simulink model "MPC_sim_sol"  (R2023b)
settings: Solver=FixedStepDiscrete  StartTime=0.0  StopTime=40  FixedStep=1  RelTol=1e-3
values from neighbouring files (symbols this model uses):
  A = [ 0 , 1 ; 0 , 0 ]    [FDBlin_pend_par_sol.m]    (also in MPC_par_sol.m = [ 1 1 ; 0 1 ]; MPC_sol.m = [ 1 1 ; 0 1 ])
  B = [ 0 ; 1 ]    [FDBlin_pend_par_sol.m]    (also in MPC_par_sol.m; MPC_sol.m)
  H = 2*(Bb'*Qb*Bb + Rb)    [MPC_par_sol.m]    (also in MPC_sol.m; QP_primer_sol.m = 2*eye(2))
  preF = Ab'*Qb*Bb    [MPC_par_sol.m]    (also in MPC_sol.m)
  Umax = 1*ones(3,1)    [MPC_par_sol.m]    (also in MPC_sol.m)
  Umin = -1*ones(3,1)    [MPC_par_sol.m]    (also in MPC_sol.m)
  x0 = [ 10 ; 0 ]    [MPC_par_sol.m]    (also in MPC_sol.m)
settings Model: Creator=jerome  LastModifiedBy=jerome
settings SolverCC: AlgebraicLoopSolver=TrustRegion
settings DebuggingCC: UnconnectedInputMsg=warning  UnconnectedOutputMsg=warning  UnconnectedLineMsg=warning
settings ModelReferenceCC: EnableRefExpFcnMdlSchedulingChecks=on
settings RTWCC: DLArmComputeVersion=19.05

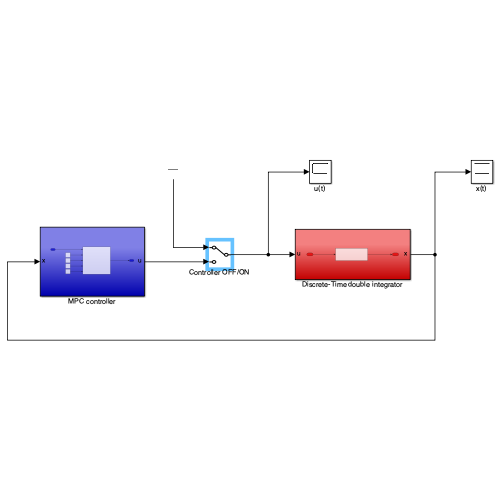
[thumbnail: Simulink's stored preview of the top-level diagram]
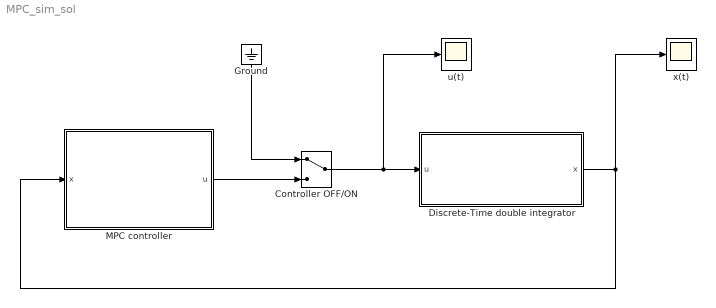
== system MPC_sim_sol ==
  Controller OFF/ON : ManualSwitch
  Discrete-Time double integrator : Subsystem
  Ground : Ground
  MPC controller : Subsystem
  u(t) : Scope
  x(t) : Scope
  wires:
  Ground/1 -> Controller OFF/ON/1
  Controller OFF/ON/1 -> Discrete-Time double integrator/1(u), u(t)/1
  Discrete-Time double integrator/1(x) -> x(t)/1, MPC controller/1(x)
  MPC controller/1(u) -> Controller OFF/ON/2

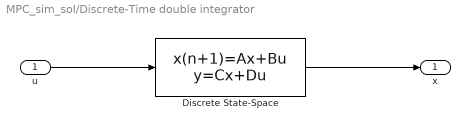
== system MPC_sim_sol/Discrete-Time double integrator ==
  u : Inport
  Discrete State-Space : DiscreteStateSpace  A=A  B=B  C=eye(2)  D=zeros(2,1)  InitialCondition=x0  SampleTime=-1
  x : Outport
  wires:
  Discrete State-Space/1 -> x/1
  u/1 -> Discrete State-Space/1

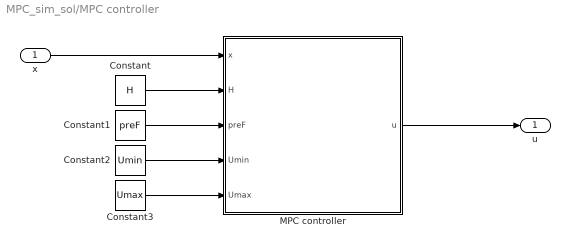
== system MPC_sim_sol/MPC controller ==
  x : Inport
  Constant : Constant  Value=H  VectorParams1D=off
  Constant1 : Constant  Value=preF  VectorParams1D=off
  Constant2 : Constant  Value=Umin  VectorParams1D=off
  Constant3 : Constant  Value=Umax  VectorParams1D=off
  MPC controller : MATLAB Function  TreatAsAtomicUnit=on
  u : Outport
  wires:
  x/1 -> MPC controller/1(x)
  Constant3/1 -> MPC controller/5(Umax)
  Constant/1 -> MPC controller/2(H)
  Constant2/1 -> MPC controller/4(Umin)
  MPC controller/1(u) -> u/1
  Constant1/1 -> MPC controller/3(preF)

== matlab function MPC_sim_sol/MPC controller/MPC controller ==
  data: x input; u output; H input; preF input; Umin input; Umax input
function u = fcn(x,H,preF,Umin,Umax)


% compute F matrix using preF matrix (defined offline)
F = (2*x'*preF)';

% make sure result of optimization is not displayed
options = optimoptions('quadprog','Display','off','Algorithm','active-set');

% compute optimal vector Ustar
Ustar = quadprog(H,F,[],[],[],[],Umin,Umax,zeros(3,1),options);
% select current input
u = Ustar(1,1);
